simulink model "Linear_Model"  (R2014b)
settings: Solver=ode45  StartTime=0.0  StopTime=600  RelTol=1e-6
settings Model: Creator=NagyZe  LastModifiedBy=NagyZe

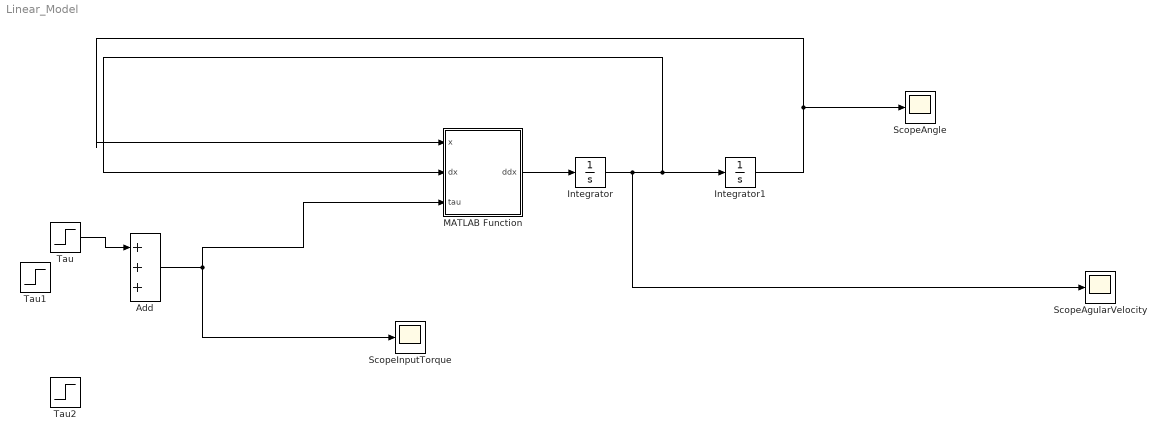
== system Linear_Model ==
  Add : Sum  Inputs=+++
  Integrator : Integrator  InitialCondition=[0 0 0]
  Integrator1 : Integrator  InitialCondition=[0 pi-0.1 0.1]
  MATLAB Function : MATLAB Function  TreatAsAtomicUnit=on
  ScopeAgularVelocity : Scope
      settings: SaveName=jointVelocity
  ScopeAngle : Scope
      settings: SaveName=jointVelocity1
  ScopeInputTorque : Scope
      settings: SaveName=jointVelocity2
  Tau : Step  Before=[0 0 0]  After=[0 0 0]  SampleTime=0
  Tau1 : Step  Time=80  Before=[0 0 0]  After=[-0.1 0 0]  SampleTime=0
  Tau2 : Step  Time=81  Before=[0 0 0]  After=[0.1 0 0]  SampleTime=0
  wires:
  MATLAB Function/1(ddx) -> Integrator/1
  Integrator/1 -> ScopeAgularVelocity/1, MATLAB Function/2(dx), Integrator1/1
  Integrator1/1 -> ScopeAngle/1, MATLAB Function/1(x)
  Add/1 -> ScopeInputTorque/1, MATLAB Function/3(tau)
  Tau/1 -> Add/1

== matlab function Linear_Model/MATLAB Function ==
  data: x input; ddx output; dx input; tau input
function ddx = fcn(x,dx,tau)
%getting the state spacemodel of the system
%give real values to the angles and the angular velocities

%giving the points where we want to liearize the system
% LINEARIZATION POINTS
% angles
q01=0;
q02=pi;
q03=0;
% angular velocities
dq01=0;
dq02=0;
dq03=0;
%angular acceleration
ddq01=0;
ddq02=0;
ddq03=0;

%giving some random data for M, L, I
L1=1.25;
L2=1.04;
L3=1.4;
M1=0.91; M2=0.61; M3=0.4;
I1x=1.1; I1y=1.2;I1z=1.3;
I2x=1; I2y=1.1; I2z=1.2;
I3x=1.2; I3y=1; I3z=1.1;
g=9.8;


q1=x(1);
q2=x(2);
q3=x(3);

dq1=dx(1);
dq2=dx(2);
dq3=dx(3);

M=[ I1z + cos(q02)*(sin(q03)*((M3*cos(q02)*sin(q03)*L3^2)/4 + I3y*cos(q02)*sin(q03)) + I2x*cos(q02) + I3x*cos(q02)*cos(q03)^2) + sin(q02)*(I2y*sin(q02) + I3z*sin(q02) + (L2^2*M2*sin(q02))/4 + (L3*M3*((L3*sin(q02))/2 + L2*cos(q03)*sin(q02)))/2 + L2*M3*cos(q03)*((L3*sin(q02))/2 + L2*cos(q03)*sin(q02)) + L2^2*M3*sin(q02)*sin(q03)^2),                                  cos(q02)*(sin(q03)*(I3y*cos(q03) + (L3*M3*(L2 + (L3*cos(q03))/2))/2) - I3x*cos(q03)*sin(q03)), -sin(q02)*((M3*L3^2)/4 + (L2*M3*cos(q03)*L3)/2 + I3z)
                                                                                                                                                                                                      cos(q03)*((M3*cos(q02)*sin(q03)*L3^2)/4 + I3y*cos(q02)*sin(q03)) - I3x*cos(q02)*cos(q03)*sin(q03) + (L2*L3*M3*cos(q02)*sin(q03))/2, I2z + cos(q03)*(I3y*cos(q03) + (L3*M3*(L2 + (L3*cos(q03))/2))/2) + (L2^2*M2)/4 + I3x*sin(q03)^2 + L2*M3*(L2 + (L3*cos(q03))/2),                                                     0
                                                                                                                                                                                                                                                                     - I3z*sin(q02) - (L3*M3*((L3*sin(q02))/2 + L2*cos(q03)*sin(q02)))/2,                                                                                                                              0,                                     (M3*L3^2)/4 + I3z];

C=zeros(3);

B =[ sin(q02)*((L3*M3*((L3*dq03*cos(q02))/2 - 2*L2*dq01*sin(q02)^2*sin(q03) + L2*dq02*cos(q02)*cos(q03) + (L3*cos(q02)*cos(q03)*(dq02*cos(q03) + dq01*cos(q02)*sin(q03)))/2 - (L3*cos(q02)*sin(q03)*(dq02*sin(q03) - dq01*cos(q02)*cos(q03)))/2))/2 - I2x*dq02*cos(q02) + I2z*dq02*cos(q02) + I3z*dq03*cos(q02) + L2*M3*sin(q03)*(2*L2*dq01*cos(q03)*sin(q02)^2 - (L3*(2*sin(q02)*(dq03 - dq01*sin(q02)) - 2*cos(q02)*sin(q03)*(dq02*cos(q03) + dq01*cos(q02)*sin(q03))))/2 + L2*dq02*cos(q02)*sin(q03)) + (L2^2*M2*dq02*cos(q02))/4 + L2*M3*cos(q03)*((L3*dq03*cos(q02))/2 - 2*L2*dq01*sin(q02)^2*sin(q03) + L2*dq02*cos(q02)*cos(q03) + (L3*cos(q02)*cos(q03)*(dq02*cos(q03) + dq01*cos(q02)*sin(q03)))/2 - (L3*cos(q02)*sin(q03)*(dq02*sin(q03) - dq01*cos(q02)*cos(q03)))/2) - I3x*cos(q02)*cos(q03)*(dq02*cos(q03) + dq01*cos(q02)*sin(q03)) + I3y*cos(q02)*cos(q03)*(dq02*cos(q03) + dq01*cos(q02)*sin(q03)) + I3x*cos(q02)*sin(q03)*(dq02*sin(q03) - dq01*cos(q02)*cos(q03)) - I3y*cos(q02)*sin(q03)*(dq02*sin(q03) - dq01*cos(q02)*cos(q03))) - cos(q02)*(sin(q03)*(I3x*sin(q02)*(dq02*sin(q03) - dq01*cos(q02)*cos(q03)) - I3z*sin(q02)*(dq02*sin(q03) - dq01*cos(q02)*cos(q03)) - (L3*M3*((L3*sin(q02)*(dq02*sin(q03) - dq01*cos(q02)*cos(q03)))/2 + (L3*cos(q02)*cos(q03)*(dq03 - dq01*sin(q02)))/2 - 2*L2*dq01*cos(q02)*sin(q02) - (L3*dq03*sin(q02)*sin(q03))/2))/2 + I3x*cos(q02)*cos(q03)*(dq03 - dq01*sin(q02)) - I3z*cos(q02)*cos(q03)*(dq03 - dq01*sin(q02)) + I3y*dq03*sin(q02)*sin(q03)) + cos(q03)*(I3y*sin(q02)*(dq02*cos(q03) + dq01*cos(q02)*sin(q03)) - I3z*sin(q02)*(dq02*cos(q03) + dq01*cos(q02)*sin(q03)) + I3x*dq03*cos(q03)*sin(q02) - I3y*cos(q02)*sin(q03)*(dq03 - dq01*sin(q02)) + I3z*cos(q02)*sin(q03)*(dq03 - dq01*sin(q02))) - I2y*dq02*sin(q02) + I2z*dq02*sin(q02)), sin(q02)*(I3x*sin(q03)*(dq02*cos(q03) + dq01*cos(q02)*sin(q03)) - I3y*sin(q03)*(dq02*cos(q03) + dq01*cos(q02)*sin(q03)) - I2x*dq01*cos(q02) + I2z*dq01*cos(q02) + I3x*cos(q03)*(dq02*sin(q03) - dq01*cos(q02)*cos(q03)) - I3y*cos(q03)*(dq02*sin(q03) - dq01*cos(q02)*cos(q03)) - (L3*M3*((L3*sin(q03)*(dq02*cos(q03) + dq01*cos(q02)*sin(q03)))/2 + 2*L2*dq02*sin(q03) + (L3*cos(q03)*(dq02*sin(q03) - dq01*cos(q02)*cos(q03)))/2 - L2*dq01*cos(q02)*cos(q03)))/2 + (L2^2*M2*dq01*cos(q02))/4 - L2*M3*cos(q03)*((L3*sin(q03)*(dq02*cos(q03) + dq01*cos(q02)*sin(q03)))/2 + 2*L2*dq02*sin(q03) + (L3*cos(q03)*(dq02*sin(q03) - dq01*cos(q02)*cos(q03)))/2 - L2*dq01*cos(q02)*cos(q03)) + L2*M3*sin(q03)*(2*L2*dq02*cos(q03) + L3*cos(q03)*(dq02*cos(q03) + dq01*cos(q02)*sin(q03)) + L2*dq01*cos(q02)*sin(q03))) - cos(q02)*(sin(q03)*((M3*sin(q03)*(dq03 - dq01*sin(q02))*L3^2)/4 - I3x*sin(q03)*(dq03 - dq01*sin(q02)) + I3z*sin(q03)*(dq03 - dq01*sin(q02))) - cos(q03)*(I3y*cos(q03)*(dq03 - dq01*sin(q02)) - I3z*cos(q03)*(dq03 - dq01*sin(q02))) - I2y*dq01*sin(q02) + I2z*dq01*sin(q02)), sin(q02)*(I3z*dq01*cos(q02) + (L3^2*M3*dq01*cos(q02))/4 + (L2*L3*M3*sin(q03)*(2*dq03 - 2*dq01*sin(q02)))/2 + (L2*L3*M3*dq01*cos(q02)*cos(q03))/2) - cos(q02)*(sin(q03)*(I3z*(dq02*sin(q03) - dq01*cos(q02)*cos(q03)) - I3x*(dq02*sin(q03) - dq01*cos(q02)*cos(q03)) + (L3*M3*((L3*(dq02*sin(q03) - dq01*cos(q02)*cos(q03)))/2 + (L3*dq01*sin(q02)*sin(q03))/2))/2 + I3y*dq01*sin(q02)*sin(q03)) + cos(q03)*(I3z*(dq02*cos(q03) + dq01*cos(q02)*sin(q03)) - I3y*(dq02*cos(q03) + dq01*cos(q02)*sin(q03)) + I3x*dq01*cos(q03)*sin(q02)))
                                                                                                                                                                                                                                                                                                                                                                                                                                                                                                                                                                                                                                                                                                                                                                                                                 sin(q03)*(I3y*sin(q02)*(dq02*cos(q03) + dq01*cos(q02)*sin(q03)) - I3z*sin(q02)*(dq02*cos(q03) + dq01*cos(q02)*sin(q03)) + I3x*dq03*cos(q03)*sin(q02) - I3y*cos(q02)*sin(q03)*(dq03 - dq01*sin(q02)) + I3z*cos(q02)*sin(q03)*(dq03 - dq01*sin(q02))) - cos(q03)*(I3x*sin(q02)*(dq02*sin(q03) - dq01*cos(q02)*cos(q03)) - I3z*sin(q02)*(dq02*sin(q03) - dq01*cos(q02)*cos(q03)) - (L3*M3*((L3*sin(q02)*(dq02*sin(q03) - dq01*cos(q02)*cos(q03)))/2 + (L3*cos(q02)*cos(q03)*(dq03 - dq01*sin(q02)))/2 - 2*L2*dq01*cos(q02)*sin(q02) - (L3*dq03*sin(q02)*sin(q03))/2))/2 + I3x*cos(q02)*cos(q03)*(dq03 - dq01*sin(q02)) - I3z*cos(q02)*cos(q03)*(dq03 - dq01*sin(q02)) + I3y*dq03*sin(q02)*sin(q03)) + L2*M3*((L3*sin(q02)*(dq02*sin(q03) - dq01*cos(q02)*cos(q03)))/2 + (L3*cos(q02)*cos(q03)*(dq03 - dq01*sin(q02)))/2 - 2*L2*dq01*cos(q02)*sin(q02) - (L3*dq03*sin(q02)*sin(q03))/2) + 2*I2x*dq01*cos(q02)*sin(q02) - 2*I2y*dq01*cos(q02)*sin(q02) - (L2^2*M2*dq01*cos(q02)*sin(q02))/2,                                                                                                                                                                                                                                                                                                                                                                                                                                                                                                                                                                                                                                                                                                                                                                                                                      - cos(q03)*((M3*sin(q03)*(dq03 - dq01*sin(q02))*L3^2)/4 - I3x*sin(q03)*(dq03 - dq01*sin(q02)) + I3z*sin(q03)*(dq03 - dq01*sin(q02))) - sin(q03)*(I3y*cos(q03)*(dq03 - dq01*sin(q02)) - I3z*cos(q03)*(dq03 - dq01*sin(q02))) - (L2*L3*M3*sin(q03)*(dq03 - dq01*sin(q02)))/2,                                                                      sin(q03)*(I3z*(dq02*cos(q03) + dq01*cos(q02)*sin(q03)) - I3y*(dq02*cos(q03) + dq01*cos(q02)*sin(q03)) + I3x*dq01*cos(q03)*sin(q02)) - cos(q03)*(I3z*(dq02*sin(q03) - dq01*cos(q02)*cos(q03)) - I3x*(dq02*sin(q03) - dq01*cos(q02)*cos(q03)) + (L3*M3*((L3*(dq02*sin(q03) - dq01*cos(q02)*cos(q03)))/2 + (L3*dq01*sin(q02)*sin(q03))/2))/2 + I3y*dq01*sin(q02)*sin(q03)) - L2*M3*((L3*(dq02*sin(q03) - dq01*cos(q02)*cos(q03)))/2 + (L3*dq01*sin(q02)*sin(q03))/2)
                                                                                                                                                                                                                                                                                                                                                                                                                                                                                                                                                                                                                                                                                                                                                                                                                                                                                                                                                                                                                                                                                                                                                                                                                                                                           I3x*cos(q02)*cos(q03)*(dq02*cos(q03) + dq01*cos(q02)*sin(q03)) - I3z*dq03*cos(q02) - (L3*M3*((L3*dq03*cos(q02))/2 - 2*L2*dq01*sin(q02)^2*sin(q03) + L2*dq02*cos(q02)*cos(q03) + (L3*cos(q02)*cos(q03)*(dq02*cos(q03) + dq01*cos(q02)*sin(q03)))/2 - (L3*cos(q02)*sin(q03)*(dq02*sin(q03) - dq01*cos(q02)*cos(q03)))/2))/2 - I3y*cos(q02)*cos(q03)*(dq02*cos(q03) + dq01*cos(q02)*sin(q03)) - I3x*cos(q02)*sin(q03)*(dq02*sin(q03) - dq01*cos(q02)*cos(q03)) + I3y*cos(q02)*sin(q03)*(dq02*sin(q03) - dq01*cos(q02)*cos(q03)),                                                                                                                                                                                                                                                                                                                                                                                                                                                                                                                                                                                                                                                                                I3y*sin(q03)*(dq02*cos(q03) + dq01*cos(q02)*sin(q03)) - I3x*sin(q03)*(dq02*cos(q03) + dq01*cos(q02)*sin(q03)) - I3x*cos(q03)*(dq02*sin(q03) - dq01*cos(q02)*cos(q03)) + I3y*cos(q03)*(dq02*sin(q03) - dq01*cos(q02)*cos(q03)) + (L3*M3*((L3*sin(q03)*(dq02*cos(q03) + dq01*cos(q02)*sin(q03)))/2 + 2*L2*dq02*sin(q03) + (L3*cos(q03)*(dq02*sin(q03) - dq01*cos(q02)*cos(q03)))/2 - L2*dq01*cos(q02)*cos(q03)))/2,                                                                                                                                                                                                                                                                                                                                                                                                                                                                                        - I3z*dq01*cos(q02) - (L3^2*M3*dq01*cos(q02))/4];
G=[ I1z*ddq01 - ddq01*(I1z + cos(q02)*(sin(q03)*((M3*cos(q02)*sin(q03)*L3^2)/4 + I3y*cos(q02)*sin(q03)) + I2x*cos(q02) + I3x*cos(q02)*cos(q03)^2) + sin(q02)*(I2y*sin(q02) + I3z*sin(q02) + (L2^2*M2*sin(q02))/4 + (L3*M3*((L3*sin(q02))/2 + L2*cos(q03)*sin(q02)))/2 + L2*M3*cos(q03)*((L3*sin(q02))/2 + L2*cos(q03)*sin(q02)) + L2^2*M3*sin(q02)*sin(q03)^2)) + dq01*(cos(q02)*(sin(q03)*(I3x*sin(q02)*(dq02*sin(q03) - dq01*cos(q02)*cos(q03)) - I3z*sin(q02)*(dq02*sin(q03) - dq01*cos(q02)*cos(q03)) - (L3*M3*((L3*sin(q02)*(dq02*sin(q03) - dq01*cos(q02)*cos(q03)))/2 + (L3*cos(q02)*cos(q03)*(dq03 - dq01*sin(q02)))/2 - 2*L2*dq01*cos(q02)*sin(q02) - (L3*dq03*sin(q02)*sin(q03))/2))/2 + I3x*cos(q02)*cos(q03)*(dq03 - dq01*sin(q02)) - I3z*cos(q02)*cos(q03)*(dq03 - dq01*sin(q02)) + I3y*dq03*sin(q02)*sin(q03)) + cos(q03)*(I3y*sin(q02)*(dq02*cos(q03) + dq01*cos(q02)*sin(q03)) - I3z*sin(q02)*(dq02*cos(q03) + dq01*cos(q02)*sin(q03)) + I3x*dq03*cos(q03)*sin(q02) - I3y*cos(q02)*sin(q03)*(dq03 - dq01*sin(q02)) + I3z*cos(q02)*sin(q03)*(dq03 - dq01*sin(q02))) - I2y*dq02*sin(q02) + I2z*dq02*sin(q02)) - sin(q02)*((L3*M3*((L3*dq03*cos(q02))/2 - 2*L2*dq01*sin(q02)^2*sin(q03) + L2*dq02*cos(q02)*cos(q03) + (L3*cos(q02)*cos(q03)*(dq02*cos(q03) + dq01*cos(q02)*sin(q03)))/2 - (L3*cos(q02)*sin(q03)*(dq02*sin(q03) - dq01*cos(q02)*cos(q03)))/2))/2 - I2x*dq02*cos(q02) + I2z*dq02*cos(q02) + I3z*dq03*cos(q02) + L2*M3*sin(q03)*(2*L2*dq01*cos(q03)*sin(q02)^2 - (L3*(2*sin(q02)*(dq03 - dq01*sin(q02)) - 2*cos(q02)*sin(q03)*(dq02*cos(q03) + dq01*cos(q02)*sin(q03))))/2 + L2*dq02*cos(q02)*sin(q03)) + (L2^2*M2*dq02*cos(q02))/4 + L2*M3*cos(q03)*((L3*dq03*cos(q02))/2 - 2*L2*dq01*sin(q02)^2*sin(q03) + L2*dq02*cos(q02)*cos(q03) + (L3*cos(q02)*cos(q03)*(dq02*cos(q03) + dq01*cos(q02)*sin(q03)))/2 - (L3*cos(q02)*sin(q03)*(dq02*sin(q03) - dq01*cos(q02)*cos(q03)))/2) - I3x*cos(q02)*cos(q03)*(dq02*cos(q03) + dq01*cos(q02)*sin(q03)) + I3y*cos(q02)*cos(q03)*(dq02*cos(q03) + dq01*cos(q02)*sin(q03)) + I3x*cos(q02)*sin(q03)*(dq02*sin(q03) - dq01*cos(q02)*cos(q03)) - I3y*cos(q02)*sin(q03)*(dq02*sin(q03) - dq01*cos(q02)*cos(q03)))) + cos(q02)*(sin(q03)*(I3y*(ddq02*cos(q03) + ddq01*cos(q02)*sin(q03) - dq01*dq03*sin(q02)*sin(q03)) + I3x*(dq03 - dq01*sin(q02))*(dq02*sin(q03) - dq01*cos(q02)*cos(q03)) - I3z*(dq03 - dq01*sin(q02))*(dq02*sin(q03) - dq01*cos(q02)*cos(q03)) - (L3*M3*(g*sin(q02) - (L3*(ddq02*cos(q03) + ddq01*cos(q02)*sin(q03) - dq01*dq03*sin(q02)*sin(q03)))/2 - L2*ddq02 + (L3*(dq03 - dq01*sin(q02))*(dq02*sin(q03) - dq01*cos(q02)*cos(q03)))/2 + L2*dq01^2*cos(q02)*sin(q02)))/2) - cos(q03)*(I3x*(ddq02*sin(q03) - ddq01*cos(q02)*cos(q03) + dq01*dq03*cos(q03)*sin(q02)) - I3y*(dq03 - dq01*sin(q02))*(dq02*cos(q03) + dq01*cos(q02)*sin(q03)) + I3z*(dq03 - dq01*sin(q02))*(dq02*cos(q03) + dq01*cos(q02)*sin(q03))) + I2x*ddq01*cos(q02) + I2y*dq01*dq02*sin(q02) - I2z*dq01*dq02*sin(q02)) + (q02 - q2)*(sin(q02)*(sin(q03)*(I3y*(ddq02*cos(q03) + ddq01*cos(q02)*sin(q03) - dq01*dq03*sin(q02)*sin(q03)) + I3x*(dq03 - dq01*sin(q02))*(dq02*sin(q03) - dq01*cos(q02)*cos(q03)) - I3z*(dq03 - dq01*sin(q02))*(dq02*sin(q03) - dq01*cos(q02)*cos(q03)) - (L3*M3*(g*sin(q02) - (L3*(ddq02*cos(q03) + ddq01*cos(q02)*sin(q03) - dq01*dq03*sin(q02)*sin(q03)))/2 - L2*ddq02 + (L3*(dq03 - dq01*sin(q02))*(dq02*sin(q03) - dq01*cos(q02)*cos(q03)))/2 + L2*dq01^2*cos(q02)*sin(q02)))/2) - cos(q03)*(I3x*(ddq02*sin(q03) - ddq01*cos(q02)*cos(q03) + dq01*dq03*cos(q03)*sin(q02)) - I3y*(dq03 - dq01*sin(q02))*(dq02*cos(q03) + dq01*cos(q02)*sin(q03)) + I3z*(dq03 - dq01*sin(q02))*(dq02*cos(q03) + dq01*cos(q02)*sin(q03))) + I2x*ddq01*cos(q02) + I2y*dq01*dq02*sin(q02) - I2z*dq01*dq02*sin(q02)) - cos(q02)*(I3z*(ddq01*sin(q02) - ddq03 + dq01*dq03*cos(q02)) + I3x*(dq02*cos(q03) + dq01*cos(q02)*sin(q03))*(dq02*sin(q03) - dq01*cos(q02)*cos(q03)) - I3y*(dq02*cos(q03) + dq01*cos(q02)*sin(q03))*(dq02*sin(q03) - dq01*cos(q02)*cos(q03)) + (L2*M2*((L2*ddq01*sin(q02))/2 + (L2*dq01*dq02*cos(q02))/2))/2 + (L3*M3*((L3*(ddq01*sin(q02) - ddq03 + dq01*dq03*cos(q02)))/2 - sin(q03)*(L2*(dq01^2*sin(q02)^2 + dq02^2) - g*cos(q02)) + cos(q03)*(L2*ddq01*sin(q02) + L2*dq01*dq02*cos(q02)) - (L3*(dq02*cos(q03) + dq01*cos(q02)*sin(q03))*(dq02*sin(q03) - dq01*cos(q02)*cos(q03)))/2))/2 + I2y*ddq01*sin(q02) + L2*M3*sin(q03)*(cos(q03)*(L2*(dq01^2*sin(q02)^2 + dq02^2) - g*cos(q02)) + (L3*((dq03 - dq01*sin(q02))^2 + (dq02*cos(q03) + dq01*cos(q02)*sin(q03))^2))/2 + sin(q03)*(L2*ddq01*sin(q02) + L2*dq01*dq02*cos(q02))) - I2x*dq01*dq02*cos(q02) + I2z*dq01*dq02*cos(q02) + L2*M3*cos(q03)*((L3*(ddq01*sin(q02) - ddq03 + dq01*dq03*cos(q02)))/2 - sin(q03)*(L2*(dq01^2*sin(q02)^2 + dq02^2) - g*cos(q02)) + cos(q03)*(L2*ddq01*sin(q02) + L2*dq01*dq02*cos(q02)) - (L3*(dq02*cos(q03) + dq01*cos(q02)*sin(q03))*(dq02*sin(q03) - dq01*cos(q02)*cos(q03)))/2)) - sin(q02)*(I3z*(ddq01*cos(q02) - dq01*dq03*sin(q02)) + (L2*M2*((L2*ddq01*cos(q02))/2 - (L2*dq01*dq02*sin(q02))/2))/2 + (L3*M3*((L3*(ddq01*cos(q02) - dq01*dq03*sin(q02)))/2 - sin(q03)*(2*L2*cos(q02)*sin(q02)*dq01^2 + g*sin(q02)) + cos(q03)*(L2*ddq01*cos(q02) - L2*dq01*dq02*sin(q02)) - (L3*dq01*cos(q03)*sin(q02)*(dq02*cos(q03) + dq01*cos(q02)*sin(q03)))/2 + (L3*dq01*sin(q02)*sin(q03)*(dq02*sin(q03) - dq01*cos(q02)*cos(q03)))/2))/2 + I2y*ddq01*cos(q02) + I2x*dq01*dq02*sin(q02) - I2z*dq01*dq02*sin(q02) + L2*M3*sin(q03)*(cos(q03)*(2*L2*cos(q02)*sin(q02)*dq01^2 + g*sin(q02)) - (L3*(2*dq01*cos(q02)*(dq03 - dq01*sin(q02)) + 2*dq01*sin(q02)*sin(q03)*(dq02*cos(q03) + dq01*cos(q02)*sin(q03))))/2 + sin(q03)*(L2*ddq01*cos(q02) - L2*dq01*dq02*sin(q02))) + L2*M3*cos(q03)*((L3*(ddq01*cos(q02) - dq01*dq03*sin(q02)))/2 - sin(q03)*(2*L2*cos(q02)*sin(q02)*dq01^2 + g*sin(q02)) + cos(q03)*(L2*ddq01*cos(q02) - L2*dq01*dq02*sin(q02)) - (L3*dq01*cos(q03)*sin(q02)*(dq02*cos(q03) + dq01*cos(q02)*sin(q03)))/2 + (L3*dq01*sin(q02)*sin(q03)*(dq02*sin(q03) - dq01*cos(q02)*cos(q03)))/2) + I3x*dq01*cos(q03)*sin(q02)*(dq02*cos(q03) + dq01*cos(q02)*sin(q03)) - I3y*dq01*cos(q03)*sin(q02)*(dq02*cos(q03) + dq01*cos(q02)*sin(q03)) - I3x*dq01*sin(q02)*sin(q03)*(dq02*sin(q03) - dq01*cos(q02)*cos(q03)) + I3y*dq01*sin(q02)*sin(q03)*(dq02*sin(q03) - dq01*cos(q02)*cos(q03))) + cos(q02)*(cos(q03)*(I3x*(ddq01*cos(q03)*sin(q02) + dq01*dq03*cos(q02)*cos(q03)) + I3y*dq01*cos(q02)*(dq02*cos(q03) + dq01*cos(q02)*sin(q03)) - I3z*dq01*cos(q02)*(dq02*cos(q03) + dq01*cos(q02)*sin(q03)) + I3y*dq01*sin(q02)*sin(q03)*(dq03 - dq01*sin(q02)) - I3z*dq01*sin(q02)*sin(q03)*(dq03 - dq01*sin(q02))) + sin(q03)*(I3y*(ddq01*sin(q02)*sin(q03) + dq01*dq03*cos(q02)*sin(q03)) + (L3*M3*((L3*(ddq01*sin(q02)*sin(q03) + dq01*dq03*cos(q02)*sin(q03)))/2 + g*cos(q02) + L2*dq01^2*cos(q02)^2 - L2*dq01^2*sin(q02)^2 - (L3*dq01*cos(q02)*(dq02*sin(q03) - dq01*cos(q02)*cos(q03)))/2 + (L3*dq01*cos(q03)*sin(q02)*(dq03 - dq01*sin(q02)))/2))/2 + I3x*dq01*cos(q02)*(dq02*sin(q03) - dq01*cos(q02)*cos(q03)) - I3z*dq01*cos(q02)*(dq02*sin(q03) - dq01*cos(q02)*cos(q03)) - I3x*dq01*cos(q03)*sin(q02)*(dq03 - dq01*sin(q02)) + I3z*dq01*cos(q03)*sin(q02)*(dq03 - dq01*sin(q02))) + I2x*ddq01*sin(q02) - I2y*dq01*dq02*cos(q02) + I2z*dq01*dq02*cos(q02))) + sin(q02)*(I3z*(ddq01*sin(q02) - ddq03 + dq01*dq03*cos(q02)) + I3x*(dq02*cos(q03) + dq01*cos(q02)*sin(q03))*(dq02*sin(q03) - dq01*cos(q02)*cos(q03)) - I3y*(dq02*cos(q03) + dq01*cos(q02)*sin(q03))*(dq02*sin(q03) - dq01*cos(q02)*cos(q03)) + (L2*M2*((L2*ddq01*sin(q02))/2 + (L2*dq01*dq02*cos(q02))/2))/2 + (L3*M3*((L3*(ddq01*sin(q02) - ddq03 + dq01*dq03*cos(q02)))/2 - sin(q03)*(L2*(dq01^2*sin(q02)^2 + dq02^2) - g*cos(q02)) + cos(q03)*(L2*ddq01*sin(q02) + L2*dq01*dq02*cos(q02)) - (L3*(dq02*cos(q03) + dq01*cos(q02)*sin(q03))*(dq02*sin(q03) - dq01*cos(q02)*cos(q03)))/2))/2 + I2y*ddq01*sin(q02) + L2*M3*sin(q03)*(cos(q03)*(L2*(dq01^2*sin(q02)^2 + dq02^2) - g*cos(q02)) + (L3*((dq03 - dq01*sin(q02))^2 + (dq02*cos(q03) + dq01*cos(q02)*sin(q03))^2))/2 + sin(q03)*(L2*ddq01*sin(q02) + L2*dq01*dq02*cos(q02))) - I2x*dq01*dq02*cos(q02) + I2z*dq01*dq02*cos(q02) + L2*M3*cos(q03)*((L3*(ddq01*sin(q02) - ddq03 + dq01*dq03*cos(q02)))/2 - sin(q03)*(L2*(dq01^2*sin(q02)^2 + dq02^2) - g*cos(q02)) + cos(q03)*(L2*ddq01*sin(q02) + L2*dq01*dq02*cos(q02)) - (L3*(dq02*cos(q03) + dq01*cos(q02)*sin(q03))*(dq02*sin(q03) - dq01*cos(q02)*cos(q03)))/2)) + dq03*(cos(q02)*(sin(q03)*(I3z*(dq02*sin(q03) - dq01*cos(q02)*cos(q03)) - I3x*(dq02*sin(q03) - dq01*cos(q02)*cos(q03)) + (L3*M3*((L3*(dq02*sin(q03) - dq01*cos(q02)*cos(q03)))/2 + (L3*dq01*sin(q02)*sin(q03))/2))/2 + I3y*dq01*sin(q02)*sin(q03)) + cos(q03)*(I3z*(dq02*cos(q03) + dq01*cos(q02)*sin(q03)) - I3y*(dq02*cos(q03) + dq01*cos(q02)*sin(q03)) + I3x*dq01*cos(q03)*sin(q02))) - sin(q02)*(I3z*dq01*cos(q02) + (L3^2*M3*dq01*cos(q02))/4 + (L2*L3*M3*sin(q03)*(2*dq03 - 2*dq01*sin(q02)))/2 + (L2*L3*M3*dq01*cos(q02)*cos(q03))/2)) + dq02*(cos(q02)*(sin(q03)*((M3*sin(q03)*(dq03 - dq01*sin(q02))*L3^2)/4 - I3x*sin(q03)*(dq03 - dq01*sin(q02)) + I3z*sin(q03)*(dq03 - dq01*sin(q02))) - cos(q03)*(I3y*cos(q03)*(dq03 - dq01*sin(q02)) - I3z*cos(q03)*(dq03 - dq01*sin(q02))) - I2y*dq01*sin(q02) + I2z*dq01*sin(q02)) - sin(q02)*(I3x*sin(q03)*(dq02*cos(q03) + dq01*cos(q02)*sin(q03)) - I3y*sin(q03)*(dq02*cos(q03) + dq01*cos(q02)*sin(q03)) - I2x*dq01*cos(q02) + I2z*dq01*cos(q02) + I3x*cos(q03)*(dq02*sin(q03) - dq01*cos(q02)*cos(q03)) - I3y*cos(q03)*(dq02*sin(q03) - dq01*cos(q02)*cos(q03)) - (L3*M3*((L3*sin(q03)*(dq02*cos(q03) + dq01*cos(q02)*sin(q03)))/2 + 2*L2*dq02*sin(q03) + (L3*cos(q03)*(dq02*sin(q03) - dq01*cos(q02)*cos(q03)))/2 - L2*dq01*cos(q02)*cos(q03)))/2 + (L2^2*M2*dq01*cos(q02))/4 - L2*M3*cos(q03)*((L3*sin(q03)*(dq02*cos(q03) + dq01*cos(q02)*sin(q03)))/2 + 2*L2*dq02*sin(q03) + (L3*cos(q03)*(dq02*sin(q03) - dq01*cos(q02)*cos(q03)))/2 - L2*dq01*cos(q02)*cos(q03)) + L2*M3*sin(q03)*(2*L2*dq02*cos(q03) + L3*cos(q03)*(dq02*cos(q03) + dq01*cos(q02)*sin(q03)) + L2*dq01*cos(q02)*sin(q03)))) - (q03 - q3)*(cos(q02)*(cos(q03)*(I3y*(ddq02*cos(q03) + ddq01*cos(q02)*sin(q03) - dq01*dq03*sin(q02)*sin(q03)) + I3x*(dq03 - dq01*sin(q02))*(dq02*sin(q03) - dq01*cos(q02)*cos(q03)) - I3z*(dq03 - dq01*sin(q02))*(dq02*sin(q03) - dq01*cos(q02)*cos(q03)) - (L3*M3*(g*sin(q02) - (L3*(ddq02*cos(q03) + ddq01*cos(q02)*sin(q03) - dq01*dq03*sin(q02)*sin(q03)))/2 - L2*ddq02 + (L3*(dq03 - dq01*sin(q02))*(dq02*sin(q03) - dq01*cos(q02)*cos(q03)))/2 + L2*dq01^2*cos(q02)*sin(q02)))/2) - sin(q03)*(I3y*(ddq02*sin(q03) - ddq01*cos(q02)*cos(q03) + dq01*dq03*cos(q03)*sin(q02)) - I3x*(dq03 - dq01*sin(q02))*(dq02*cos(q03) + dq01*cos(q02)*sin(q03)) + I3z*(dq03 - dq01*sin(q02))*(dq02*cos(q03) + dq01*cos(q02)*sin(q03)) + (L3*M3*((L3*(ddq02*sin(q03) - ddq01*cos(q02)*cos(q03) + dq01*dq03*cos(q03)*sin(q02)))/2 + (L3*(dq03 - dq01*sin(q02))*(dq02*cos(q03) + dq01*cos(q02)*sin(q03)))/2))/2) + sin(q03)*(I3x*(ddq02*sin(q03) - ddq01*cos(q02)*cos(q03) + dq01*dq03*cos(q03)*sin(q02)) - I3y*(dq03 - dq01*sin(q02))*(dq02*cos(q03) + dq01*cos(q02)*sin(q03)) + I3z*(dq03 - dq01*sin(q02))*(dq02*cos(q03) + dq01*cos(q02)*sin(q03))) - cos(q03)*(I3x*(ddq02*cos(q03) + ddq01*cos(q02)*sin(q03) - dq01*dq03*sin(q02)*sin(q03)) + I3y*(dq03 - dq01*sin(q02))*(dq02*sin(q03) - dq01*cos(q02)*cos(q03)) - I3z*(dq03 - dq01*sin(q02))*(dq02*sin(q03) - dq01*cos(q02)*cos(q03)))) - sin(q02)*(I3x*(dq02*sin(q03) - dq01*cos(q02)*cos(q03))^2 - I3x*(dq02*cos(q03) + dq01*cos(q02)*sin(q03))^2 + I3y*(dq02*cos(q03) + dq01*cos(q02)*sin(q03))^2 - I3y*(dq02*sin(q03) - dq01*cos(q02)*cos(q03))^2 + (L3*M3*(cos(q03)*(L2*(dq01^2*sin(q02)^2 + dq02^2) - g*cos(q02)) + (L3*(dq02*cos(q03) + dq01*cos(q02)*sin(q03))^2)/2 - (L3*(dq02*sin(q03) - dq01*cos(q02)*cos(q03))^2)/2 + sin(q03)*(L2*ddq01*sin(q02) + L2*dq01*dq02*cos(q02))))/2 + L2*M3*sin(q03)*(sin(q03)*(L2*(dq01^2*sin(q02)^2 + dq02^2) - g*cos(q02)) - cos(q03)*(L2*ddq01*sin(q02) + L2*dq01*dq02*cos(q02)) + L3*(dq02*cos(q03) + dq01*cos(q02)*sin(q03))*(dq02*sin(q03) - dq01*cos(q02)*cos(q03))) - L2*M3*cos(q03)*(cos(q03)*(L2*(dq01^2*sin(q02)^2 + dq02^2) - g*cos(q02)) + (L3*((dq03 - dq01*sin(q02))^2 + (dq02*cos(q03) + dq01*cos(q02)*sin(q03))^2))/2 + sin(q03)*(L2*ddq01*sin(q02) + L2*dq01*dq02*cos(q02))) + L2*M3*cos(q03)*(cos(q03)*(L2*(dq01^2*sin(q02)^2 + dq02^2) - g*cos(q02)) + (L3*(dq02*cos(q03) + dq01*cos(q02)*sin(q03))^2)/2 - (L3*(dq02*sin(q03) - dq01*cos(q02)*cos(q03))^2)/2 + sin(q03)*(L2*ddq01*sin(q02) + L2*dq01*dq02*cos(q02))) + L2*M3*sin(q03)*((L3*(ddq01*sin(q02) - ddq03 + dq01*dq03*cos(q02)))/2 - sin(q03)*(L2*(dq01^2*sin(q02)^2 + dq02^2) - g*cos(q02)) + cos(q03)*(L2*ddq01*sin(q02) + L2*dq01*dq02*cos(q02)) - (L3*(dq02*cos(q03) + dq01*cos(q02)*sin(q03))*(dq02*sin(q03) - dq01*cos(q02)*cos(q03)))/2))) - ddq02*cos(q02)*(sin(q03)*(I3y*cos(q03) + (L3*M3*(L2 + (L3*cos(q03))/2))/2) - I3x*cos(q03)*sin(q03)) + ddq03*sin(q02)*((M3*L3^2)/4 + (L2*M3*cos(q03)*L3)/2 + I3z), dq03*(cos(q03)*(I3z*(dq02*sin(q03) - dq01*cos(q02)*cos(q03)) - I3x*(dq02*sin(q03) - dq01*cos(q02)*cos(q03)) + (L3*M3*((L3*(dq02*sin(q03) - dq01*cos(q02)*cos(q03)))/2 + (L3*dq01*sin(q02)*sin(q03))/2))/2 + I3y*dq01*sin(q02)*sin(q03)) - sin(q03)*(I3z*(dq02*cos(q03) + dq01*cos(q02)*sin(q03)) - I3y*(dq02*cos(q03) + dq01*cos(q02)*sin(q03)) + I3x*dq01*cos(q03)*sin(q02)) + L2*M3*((L3*(dq02*sin(q03) - dq01*cos(q02)*cos(q03)))/2 + (L3*dq01*sin(q02)*sin(q03))/2)) - ddq02*(I2z + cos(q03)*(I3y*cos(q03) + (L3*M3*(L2 + (L3*cos(q03))/2))/2) + (L2^2*M2)/4 + I3x*sin(q03)^2 + L2*M3*(L2 + (L3*cos(q03))/2)) + I2z*ddq02 + (q02 - q2)*(cos(q03)*(I3y*(ddq01*sin(q02)*sin(q03) + dq01*dq03*cos(q02)*sin(q03)) + (L3*M3*((L3*(ddq01*sin(q02)*sin(q03) + dq01*dq03*cos(q02)*sin(q03)))/2 + g*cos(q02) + L2*dq01^2*cos(q02)^2 - L2*dq01^2*sin(q02)^2 - (L3*dq01*cos(q02)*(dq02*sin(q03) - dq01*cos(q02)*cos(q03)))/2 + (L3*dq01*cos(q03)*sin(q02)*(dq03 - dq01*sin(q02)))/2))/2 + I3x*dq01*cos(q02)*(dq02*sin(q03) - dq01*cos(q02)*cos(q03)) - I3z*dq01*cos(q02)*(dq02*sin(q03) - dq01*cos(q02)*cos(q03)) - I3x*dq01*cos(q03)*sin(q02)*(dq03 - dq01*sin(q02)) + I3z*dq01*cos(q03)*sin(q02)*(dq03 - dq01*sin(q02))) - sin(q03)*(I3x*(ddq01*cos(q03)*sin(q02) + dq01*dq03*cos(q02)*cos(q03)) + I3y*dq01*cos(q02)*(dq02*cos(q03) + dq01*cos(q02)*sin(q03)) - I3z*dq01*cos(q02)*(dq02*cos(q03) + dq01*cos(q02)*sin(q03)) + I3y*dq01*sin(q02)*sin(q03)*(dq03 - dq01*sin(q02)) - I3z*dq01*sin(q02)*sin(q03)*(dq03 - dq01*sin(q02))) + (L2*M2*(g*cos(q02) + (L2*dq01^2*cos(q02)^2)/2 - (L2*dq01^2*sin(q02)^2)/2))/2 + L2*M3*((L3*(ddq01*sin(q02)*sin(q03) + dq01*dq03*cos(q02)*sin(q03)))/2 + g*cos(q02) + L2*dq01^2*cos(q02)^2 - L2*dq01^2*sin(q02)^2 - (L3*dq01*cos(q02)*(dq02*sin(q03) - dq01*cos(q02)*cos(q03)))/2 + (L3*dq01*cos(q03)*sin(q02)*(dq03 - dq01*sin(q02)))/2) - I2x*dq01^2*cos(q02)^2 + I2y*dq01^2*cos(q02)^2 + I2x*dq01^2*sin(q02)^2 - I2y*dq01^2*sin(q02)^2) + dq02*(cos(q03)*((M3*sin(q03)*(dq03 - dq01*sin(q02))*L3^2)/4 - I3x*sin(q03)*(dq03 - dq01*sin(q02)) + I3z*sin(q03)*(dq03 - dq01*sin(q02))) + sin(q03)*(I3y*cos(q03)*(dq03 - dq01*sin(q02)) - I3z*cos(q03)*(dq03 - dq01*sin(q02))) + (L2*L3*M3*sin(q03)*(dq03 - dq01*sin(q02)))/2) - ddq01*(cos(q03)*((M3*cos(q02)*sin(q03)*L3^2)/4 + I3y*cos(q02)*sin(q03)) - I3x*cos(q02)*cos(q03)*sin(q03) + (L2*L3*M3*cos(q02)*sin(q03))/2) + cos(q03)*(I3y*(ddq02*cos(q03) + ddq01*cos(q02)*sin(q03) - dq01*dq03*sin(q02)*sin(q03)) + I3x*(dq03 - dq01*sin(q02))*(dq02*sin(q03) - dq01*cos(q02)*cos(q03)) - I3z*(dq03 - dq01*sin(q02))*(dq02*sin(q03) - dq01*cos(q02)*cos(q03)) - (L3*M3*(g*sin(q02) - (L3*(ddq02*cos(q03) + ddq01*cos(q02)*sin(q03) - dq01*dq03*sin(q02)*sin(q03)))/2 - L2*ddq02 + (L3*(dq03 - dq01*sin(q02))*(dq02*sin(q03) - dq01*cos(q02)*cos(q03)))/2 + L2*dq01^2*cos(q02)*sin(q02)))/2) - dq01*(sin(q03)*(I3y*sin(q02)*(dq02*cos(q03) + dq01*cos(q02)*sin(q03)) - I3z*sin(q02)*(dq02*cos(q03) + dq01*cos(q02)*sin(q03)) + I3x*dq03*cos(q03)*sin(q02) - I3y*cos(q02)*sin(q03)*(dq03 - dq01*sin(q02)) + I3z*cos(q02)*sin(q03)*(dq03 - dq01*sin(q02))) - cos(q03)*(I3x*sin(q02)*(dq02*sin(q03) - dq01*cos(q02)*cos(q03)) - I3z*sin(q02)*(dq02*sin(q03) - dq01*cos(q02)*cos(q03)) - (L3*M3*((L3*sin(q02)*(dq02*sin(q03) - dq01*cos(q02)*cos(q03)))/2 + (L3*cos(q02)*cos(q03)*(dq03 - dq01*sin(q02)))/2 - 2*L2*dq01*cos(q02)*sin(q02) - (L3*dq03*sin(q02)*sin(q03))/2))/2 + I3x*cos(q02)*cos(q03)*(dq03 - dq01*sin(q02)) - I3z*cos(q02)*cos(q03)*(dq03 - dq01*sin(q02)) + I3y*dq03*sin(q02)*sin(q03)) + L2*M3*((L3*sin(q02)*(dq02*sin(q03) - dq01*cos(q02)*cos(q03)))/2 + (L3*cos(q02)*cos(q03)*(dq03 - dq01*sin(q02)))/2 - 2*L2*dq01*cos(q02)*sin(q02) - (L3*dq03*sin(q02)*sin(q03))/2) + 2*I2x*dq01*cos(q02)*sin(q02) - 2*I2y*dq01*cos(q02)*sin(q02) - (L2^2*M2*dq01*cos(q02)*sin(q02))/2) + sin(q03)*(I3x*(ddq02*sin(q03) - ddq01*cos(q02)*cos(q03) + dq01*dq03*cos(q03)*sin(q02)) - I3y*(dq03 - dq01*sin(q02))*(dq02*cos(q03) + dq01*cos(q02)*sin(q03)) + I3z*(dq03 - dq01*sin(q02))*(dq02*cos(q03) + dq01*cos(q02)*sin(q03))) + (q03 - q3)*(cos(q03)*(I3y*(ddq02*sin(q03) - ddq01*cos(q02)*cos(q03) + dq01*dq03*cos(q03)*sin(q02)) - I3x*(dq03 - dq01*sin(q02))*(dq02*cos(q03) + dq01*cos(q02)*sin(q03)) + I3z*(dq03 - dq01*sin(q02))*(dq02*cos(q03) + dq01*cos(q02)*sin(q03)) + (L3*M3*((L3*(ddq02*sin(q03) - ddq01*cos(q02)*cos(q03) + dq01*dq03*cos(q03)*sin(q02)))/2 + (L3*(dq03 - dq01*sin(q02))*(dq02*cos(q03) + dq01*cos(q02)*sin(q03)))/2))/2) + sin(q03)*(I3y*(ddq02*cos(q03) + ddq01*cos(q02)*sin(q03) - dq01*dq03*sin(q02)*sin(q03)) + I3x*(dq03 - dq01*sin(q02))*(dq02*sin(q03) - dq01*cos(q02)*cos(q03)) - I3z*(dq03 - dq01*sin(q02))*(dq02*sin(q03) - dq01*cos(q02)*cos(q03)) - (L3*M3*(g*sin(q02) - (L3*(ddq02*cos(q03) + ddq01*cos(q02)*sin(q03) - dq01*dq03*sin(q02)*sin(q03)))/2 - L2*ddq02 + (L3*(dq03 - dq01*sin(q02))*(dq02*sin(q03) - dq01*cos(q02)*cos(q03)))/2 + L2*dq01^2*cos(q02)*sin(q02)))/2) - cos(q03)*(I3x*(ddq02*sin(q03) - ddq01*cos(q02)*cos(q03) + dq01*dq03*cos(q03)*sin(q02)) - I3y*(dq03 - dq01*sin(q02))*(dq02*cos(q03) + dq01*cos(q02)*sin(q03)) + I3z*(dq03 - dq01*sin(q02))*(dq02*cos(q03) + dq01*cos(q02)*sin(q03))) - sin(q03)*(I3x*(ddq02*cos(q03) + ddq01*cos(q02)*sin(q03) - dq01*dq03*sin(q02)*sin(q03)) + I3y*(dq03 - dq01*sin(q02))*(dq02*sin(q03) - dq01*cos(q02)*cos(q03)) - I3z*(dq03 - dq01*sin(q02))*(dq02*sin(q03) - dq01*cos(q02)*cos(q03))) + L2*M3*((L3*(ddq02*sin(q03) - ddq01*cos(q02)*cos(q03) + dq01*dq03*cos(q03)*sin(q02)))/2 + (L3*(dq03 - dq01*sin(q02))*(dq02*cos(q03) + dq01*cos(q02)*sin(q03)))/2)) - (L2*M2*((L2*cos(q02)*sin(q02)*dq01^2)/2 - (L2*ddq02)/2 + g*sin(q02)))/2 - L2*M3*(g*sin(q02) - (L3*(ddq02*cos(q03) + ddq01*cos(q02)*sin(q03) - dq01*dq03*sin(q02)*sin(q03)))/2 - L2*ddq02 + (L3*(dq03 - dq01*sin(q02))*(dq02*sin(q03) - dq01*cos(q02)*cos(q03)))/2 + L2*dq01^2*cos(q02)*sin(q02)) + I2x*dq01^2*cos(q02)*sin(q02) - I2y*dq01^2*cos(q02)*sin(q02), dq01*((L3*M3*((L3*dq03*cos(q02))/2 - 2*L2*dq01*sin(q02)^2*sin(q03) + L2*dq02*cos(q02)*cos(q03) + (L3*cos(q02)*cos(q03)*(dq02*cos(q03) + dq01*cos(q02)*sin(q03)))/2 - (L3*cos(q02)*sin(q03)*(dq02*sin(q03) - dq01*cos(q02)*cos(q03)))/2))/2 + I3z*dq03*cos(q02) - I3x*cos(q02)*cos(q03)*(dq02*cos(q03) + dq01*cos(q02)*sin(q03)) + I3y*cos(q02)*cos(q03)*(dq02*cos(q03) + dq01*cos(q02)*sin(q03)) + I3x*cos(q02)*sin(q03)*(dq02*sin(q03) - dq01*cos(q02)*cos(q03)) - I3y*cos(q02)*sin(q03)*(dq02*sin(q03) - dq01*cos(q02)*cos(q03))) - dq02*(I3y*sin(q03)*(dq02*cos(q03) + dq01*cos(q02)*sin(q03)) - I3x*sin(q03)*(dq02*cos(q03) + dq01*cos(q02)*sin(q03)) - I3x*cos(q03)*(dq02*sin(q03) - dq01*cos(q02)*cos(q03)) + I3y*cos(q03)*(dq02*sin(q03) - dq01*cos(q02)*cos(q03)) + (L3*M3*((L3*sin(q03)*(dq02*cos(q03) + dq01*cos(q02)*sin(q03)))/2 + 2*L2*dq02*sin(q03) + (L3*cos(q03)*(dq02*sin(q03) - dq01*cos(q02)*cos(q03)))/2 - L2*dq01*cos(q02)*cos(q03)))/2) - I3z*(ddq01*sin(q02) - ddq03 + dq01*dq03*cos(q02)) + dq03*((M3*dq01*cos(q02)*L3^2)/4 + I3z*dq01*cos(q02)) - ddq03*((M3*L3^2)/4 + I3z) - (q03 - q3)*(I3x*(dq02*sin(q03) - dq01*cos(q02)*cos(q03))^2 - I3x*(dq02*cos(q03) + dq01*cos(q02)*sin(q03))^2 + I3y*(dq02*cos(q03) + dq01*cos(q02)*sin(q03))^2 - I3y*(dq02*sin(q03) - dq01*cos(q02)*cos(q03))^2 + (L3*M3*(cos(q03)*(L2*(dq01^2*sin(q02)^2 + dq02^2) - g*cos(q02)) + (L3*(dq02*cos(q03) + dq01*cos(q02)*sin(q03))^2)/2 - (L3*(dq02*sin(q03) - dq01*cos(q02)*cos(q03))^2)/2 + sin(q03)*(L2*ddq01*sin(q02) + L2*dq01*dq02*cos(q02))))/2) + (q02 - q2)*(I3z*(ddq01*cos(q02) - dq01*dq03*sin(q02)) + (L3*M3*((L3*(ddq01*cos(q02) - dq01*dq03*sin(q02)))/2 - sin(q03)*(2*L2*cos(q02)*sin(q02)*dq01^2 + g*sin(q02)) + cos(q03)*(L2*ddq01*cos(q02) - L2*dq01*dq02*sin(q02)) - (L3*dq01*cos(q03)*sin(q02)*(dq02*cos(q03) + dq01*cos(q02)*sin(q03)))/2 + (L3*dq01*sin(q02)*sin(q03)*(dq02*sin(q03) - dq01*cos(q02)*cos(q03)))/2))/2 + I3x*dq01*cos(q03)*sin(q02)*(dq02*cos(q03) + dq01*cos(q02)*sin(q03)) - I3y*dq01*cos(q03)*sin(q02)*(dq02*cos(q03) + dq01*cos(q02)*sin(q03)) - I3x*dq01*sin(q02)*sin(q03)*(dq02*sin(q03) - dq01*cos(q02)*cos(q03)) + I3y*dq01*sin(q02)*sin(q03)*(dq02*sin(q03) - dq01*cos(q02)*cos(q03))) + ddq01*(I3z*sin(q02) + (L3*M3*((L3*sin(q02))/2 + L2*cos(q03)*sin(q02)))/2) - I3x*(dq02*cos(q03) + dq01*cos(q02)*sin(q03))*(dq02*sin(q03) - dq01*cos(q02)*cos(q03)) + I3y*(dq02*cos(q03) + dq01*cos(q02)*sin(q03))*(dq02*sin(q03) - dq01*cos(q02)*cos(q03)) - (L3*M3*((L3*(ddq01*sin(q02) - ddq03 + dq01*dq03*cos(q02)))/2 - sin(q03)*(L2*(dq01^2*sin(q02)^2 + dq02^2) - g*cos(q02)) + cos(q03)*(L2*ddq01*sin(q02) + L2*dq01*dq02*cos(q02)) - (L3*(dq02*cos(q03) + dq01*cos(q02)*sin(q03))*(dq02*sin(q03) - dq01*cos(q02)*cos(q03)))/2))/2]';


dx=[dx(1) dx(2) dx(3)]';
%evaluating the matrices

%ddx = - inv(M)*C*dx.^2 - M\B*dx + M\tau; 

ddx = - inv(M)*C*dx.^2 - M\B*dx -M\G + M\tau; 


end
